simulink model "queuetest"  (R2018a)
settings: Solver=FixedStepDiscrete  StartTime=0.0  StopTime=inf  RelTol=1e-3  EnableMultiTasking=on
libraries: dspsigops x2, dspmisc x1, dspbuff3 x1
settings Model: ExtModeTrigMode=oneshot  ExtModeArmWhenConnect=off  Creator=The MathWorks, Inc.  LastModifiedBy=Michael Girbino
settings DataIOCC: SaveFormat=Array  SaveOutput=off  SaveTime=off
settings OptimizationCC: BlockReduction=off  BooleanDataType=off  ExpressionDepthLimit=2147483647  InitFltsAndDblsToZero=on  LifeSpan=inf  BufferReusableBoundary=off  SimCompilerOptimization=on
settings DebuggingCC: UnderspecifiedInitializationDetection=Classic  MergeDetectMultiDrivingBlocksExec=none  SignalResolutionControl=TryResolveAllWithWarning  MultiTaskDSMMsg=warning  MultiTaskCondExecSysMsg=none  IntegerOverflowMsg=none  FcnCallInpInsideContextMsg=warning  BusObjectLabelMismatch=none  StateNameClashWarn=warning  SFUnexpectedBacktrackingDiag=warning  SFNoUnconditionalDefaultTransitionDiag=warning  SFExecutionAtInitializationDiag=none  IntegerSaturationMsg=none
settings HardwareCC: ProdBitPerPointer=32  ProdBitPerSizeT=32  ProdBitPerPtrDiffT=32  ProdLargestAtomicFloat=None  ProdIntDivRoundTo=Undefined  ProdEndianess=Unspecified  ProdWordSize=32  ProdHWDeviceType=32-bit Generic  TargetUnknown=on
settings ModelReferenceCC: PropagateSignalLabelsOutOfModel=off
settings RTWCC: Description=Generic Real-Time Target  RetainRTWFile=on
settings CodeAppCC: StateflowObjectComments=on
settings GRTTargetCC: TargetLangStandard=C89/C90 (ANSI)  GeneratePreprocessorConditionals=Disable all  CombineOutputUpdateFcns=off  GRTInterface=on
settings ConfigComp: CovMetricSettings=dw  CovHtmlReporting=on  CovSaveCumulativeToWorkspaceVar=on  CovSaveSingleToWorkspaceVar=on  CovExternalEMLEnable=off  CovSFcnEnable=off

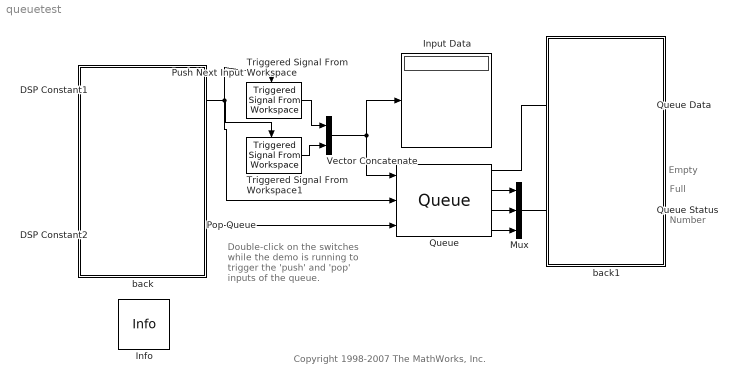
== system queuetest ==
  note: Number
  note: Full
  note: Empty
  note: Double-click on the switches
      | while the demo is running
      | to trigger the 'push' and 'pop'
      | inputs of the queue.
  note: Copyright 1998-2007 The MathWorks, Inc.
  DSP Constant1 : Constant  SampleTime=4
  DSP Constant2 : Constant  Value=0  SampleTime=4
  Info : dspmisc/Info  SystemSampleTime=-1
      settings: SourceProductName=DSP System Toolbox  SourceProductBaseCode=DS
  Input Data : Display
  Mux : Mux  Inputs=3
  Pop Queue : ManualSwitch  CurrentSetting=0
  Push Next Input : ManualSwitch  CurrentSetting=0
  Queue : dspbuff3/Queue  depth=3  trigger=Either edge  overflow=Warning  pes=Warning  eso=on  fso=on  nso=on  clr=off  clrOutport=on  adf=on
      settings: SourceProductName=DSP System Toolbox  SourceProductBaseCode=DS
  Queue Data : Display
  Queue Status : Display
  Triggered Signal From Workspace : dspsigops/Triggered Signal From Workspace  Signal=1:32  TriggerType=Either edge  ic=0  SamplesPerFrame=1  OutputAfterFinalValue=Setting to zero  OutputFrames=off
      settings: SourceProductName=DSP System Toolbox  SourceProductBaseCode=DS
  Triggered Signal From Workspace1 : dspsigops/Triggered Signal From Workspace  Signal=4:36  TriggerType=Either edge  ic=0  SamplesPerFrame=1  OutputAfterFinalValue=Setting to zero  OutputFrames=off
      settings: SourceProductName=DSP System Toolbox  SourceProductBaseCode=DS
  Vector Concatenate : Concatenate
  back : Subsystem
  back1 : Subsystem
  wires:
  Pop Queue/1 -> Queue/3
  Queue/3 -> Mux/2
  Queue/2 -> Mux/1
  Queue/4 -> Mux/3
  Mux/1 -> Queue Status/1
  Push Next Input/1 -> Triggered Signal From Workspace1/Trigger, Queue/2, Triggered Signal From Workspace/Trigger
  DSP Constant1/1 -> Pop Queue/1, Push Next Input/1
  DSP Constant2/1 -> Pop Queue/2, Push Next Input/2
  Queue/1 -> Queue Data/1
  Triggered Signal From Workspace/1 -> Vector Concatenate/1
  Vector Concatenate/1 -> Queue/1, Input Data/1
  Triggered Signal From Workspace1/1 -> Vector Concatenate/2

== system queuetest/back ==

== system queuetest/back1 ==
